simulink model "GATE_A"  (R2016a)
settings: Solver=FixedStepDiscrete  StartTime=0.0  StopTime=120  RelTol=1e-3
values from neighbouring files (symbols this model uses):
  CLOSE_CHAR = CHAR_STAR    [GateParameter.m]
  CLOSE_SIDE_VALUE = single(4*ONE_SEC)    [GateParameter.m]
  CLOSED = uint8(12)    [GateParameter.m]
  CLOSING = uint8(13)    [GateParameter.m]
  INIT = uint8(15)    [GateParameter.m]
  NO_PASS_ASSIG = uint8(6)    [GateParameter.m]
  OPEN = uint8(14)    [GateParameter.m]
  OPEN_CHAR = CHAR_HASH    [GateParameter.m]
  OPEN_SIDE_VALUE = uint16(4*ONE_SEC)    [GateParameter.m]
  OPENING = uint8(11)    [GateParameter.m]
  OPENING_ACTIVE = uint8(1)    [GateParameter.m]
  PASS_ASSIGNED = uint8(7)    [GateParameter.m]
  PASS_INCOMPLETE = uint8(8)    [GateParameter.m]
  PASS_TIMEOUT = uint16(10*ONE_SEC)    [GateParameter.m]
  PASSWORD_VERIFIED = uint8(5)    [GateParameter.m]
  TIMEOUT = uint8(9)    [GateParameter.m]
  WRONG_PASSWORD = uint8(2)    [GateParameter.m]
undefined symbols (not defined in the file or in its folder): OPEN_TIMEOUT
(part 1 of 2)
settings Model: ExtModeTrigDuration=2  Creator=omaro  LastModifiedBy=oelkawok
settings DataIOCC: SaveFormat=StructureWithTime  SaveOutput=off  SaveTime=off
settings OptimizationCC: DefaultParameterBehavior=Inlined  StateBitsets=on  DataBitsets=on  LifeSpan=1  MaxStackSize=64
settings DebuggingCC: ConsistencyChecking=error  SignalInfNanChecking=error  SignalRangeChecking=error  ReadBeforeWriteMsg=EnableAllAsError  WriteAfterWriteMsg=EnableAllAsError  WriteAfterReadMsg=EnableAllAsError  AlgebraicLoopMsg=error  ArtificialAlgebraicLoopMsg=error  BlockPriorityViolationMsg=error  MinStepSizeMsg=error  CheckMatrixSingularityMsg=error  ParameterUnderflowMsg=error  ParameterPrecisionLossMsg=error  UnderSpecifiedDataTypeMsg=warning  UnnecessaryDatatypeConvMsg=warning  VectorMatrixConversionMsg=error  SignalLabelMismatchMsg=error  UnconnectedInputMsg=error  UnconnectedOutputMsg=error  UnconnectedLineMsg=error  SFcnCompatibilityMsg=error  UniqueDataStoreMsg=error  BusObjectLabelMismatch=error  RootOutportRequireBusObject=error  ModelReferenceIOMsg=error  ModelReferenceVersionMismatchMessage=warning  ModelReferenceIOMismatchMessage=error  ModelReferenceDataLoggingMessage=error  StrictBusMsg=ErrorOnBusTreatedAsVector  SFUnusedDataAndEventsDiag=error  SFUnexpectedBacktrackingDiag=error  SFInvalidInputDataAccessInChartInitDiag=error  SFNoUnconditionalDefaultTransitionDiag=error  SFTransitionOutsideNaturalParentDiag=error  SFUndirectedBroadcastEventsDiag=error  SFTransitionActionBeforeConditionDiag=error  SFOutputUsedAsStateInMooreChartDiag=warning
settings HardwareCC: ProdBitPerInt=16  ProdBitPerPointer=16  ProdLargestAtomicFloat=None  ProdWordSize=8  ProdHWDeviceType=Atmel->AVR
settings SFSimCC: SimCustomHeaderCode=|
  | //#include "C:\Users\omaro\Desktop\Gate_Model\Arduino\Arduino.h"
  | //#include "Keypad\Keypad.h"
settings RTWCC: SystemTargetFile=ert.tlc  TemplateMakefile=ert_default_tmf  GenerateReport=on  RTWUseSimCustomCode=on  Toolchain=Arduino AVR v1.6.1  BuildConfiguration=Faster Runs  LaunchReport=on
settings RTWCC: CustomHeaderCode=|
  | //#include "C:\Users\omaro\Desktop\Gate_Model\Arduino\Arduino.h"
  | //#include "Keypad\Keypad.h"
settings CodeAppCC: ForceParamTrailComments=on  OperatorAnnotations=on  MATLABSourceComments=on
settings ERTTargetCC: ERTCustomFileBanners=off  SupportContinuousTime=on  SupportNonInlinedSFcns=on  SupportVariableSizeSignals=on  ModelStepFunctionPrototypeControlCompliant=off  RootIOFormat=Structure reference  ERTCustomFileTemplate=example_file_process.tlc

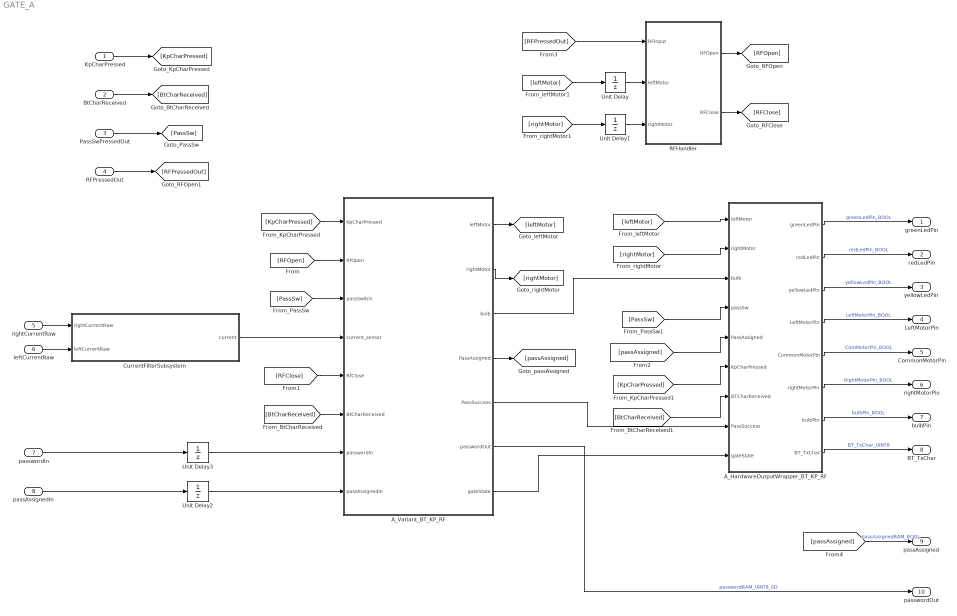
== system GATE_A ==
  KpCharPressed : Inport  OutDataTypeStr=uint8  PortDimensions=1  SampleTime=0
  BtCharReceived : Inport  Port=2  OutDataTypeStr=uint8  PortDimensions=1  SampleTime=0
  PassSwPressedOut : Inport  Port=3  OutDataTypeStr=boolean  PortDimensions=1  SampleTime=0
  RFPressedOut : Inport  Port=4  OutDataTypeStr=uint8  PortDimensions=1  SampleTime=0
  rightCurrentRaw : Inport  Port=5  OutDataTypeStr=uint16  PortDimensions=1  SampleTime=0
  leftCurrentRaw : Inport  Port=6  OutDataTypeStr=uint16  PortDimensions=1  SampleTime=0
  passwordIn : Inport  Port=7  OutDataTypeStr=uint8  PortDimensions=6  SampleTime=0
  passAssignedIn : Inport  Port=8  OutDataTypeStr=boolean  PortDimensions=1  SampleTime=0
  A_HardwareOutputWrapper_BT_KP_RF : Subsystem  VariantControl=Variant1
  A_Variant_BT_KP_RF : Subsystem  VariantControl=Variant
  CurrentFilterSubsystem : Subsystem
  RFHandler : Subsystem
  Unit Delay{,1..3} (4 alike) : UnitDelay  SampleTime=-1
  greenLedPin : Outport  OutDataTypeStr=boolean  PortDimensions=1  SampleTime=[0.001,0]
  redLedPin : Outport  Port=2  OutDataTypeStr=boolean  PortDimensions=1  SampleTime=[0.001,0]
  yellowLedPin : Outport  Port=3  OutDataTypeStr=boolean  PortDimensions=1  SampleTime=[0.001,0]
  LeftMotorPin : Outport  Port=4  OutDataTypeStr=boolean  PortDimensions=1  SampleTime=[0.001,0]
  CommonMotorPin : Outport  Port=5  OutDataTypeStr=boolean  PortDimensions=1  SampleTime=[0.001,0]
  rightMotorPin : Outport  Port=6  OutDataTypeStr=boolean  PortDimensions=1  SampleTime=[0.001,0]
  bulbPin : Outport  Port=7  OutDataTypeStr=boolean  PortDimensions=1  SampleTime=[0.001,0]
  BT_TxChar : Outport  Port=8  OutDataTypeStr=uint8  PortDimensions=1  SampleTime=[0.001,0]
  passAssigned : Outport  Port=9  OutDataTypeStr=boolean  PortDimensions=1  SampleTime=[0.001,0]
  passwordOut : Outport  Port=10  OutDataTypeStr=uint8  PortDimensions=6  SampleTime=[0.001,0]
  wires:
  RFHandler/1(RFOpen) -> [RFOpen]
  RFHandler/2(RFClose) -> [RFClose]
  [RFPressedOut] -> RFHandler/1(RFInput)
  RFPressedOut/1 -> [RFPressedOut]
  PassSwPressedOut/1 -> [PassSw]
  [leftMotor] -> Unit Delay/1
  Unit Delay/1 -> RFHandler/2(leftMotor)
  [rightMotor] -> Unit Delay1/1
  Unit Delay1/1 -> RFHandler/3(rightMotor)
  BtCharReceived/1 -> [BtCharReceived]
  KpCharPressed/1 -> [KpCharPressed]
  [RFOpen] -> A_Variant_BT_KP_RF/2(RfOpen)
  [PassSw] -> A_Variant_BT_KP_RF/3(passSwitch)
  [RFClose] -> A_Variant_BT_KP_RF/5(RfClose)
  [BtCharReceived] -> A_Variant_BT_KP_RF/6(BtCharReceived)
  A_Variant_BT_KP_RF/1(leftMotor) -> [leftMotor]
  A_Variant_BT_KP_RF/2(rightMotor) -> [rightMotor]
  [KpCharPressed] -> A_Variant_BT_KP_RF/1(KpCharPressed)
  [leftMotor] -> A_HardwareOutputWrapper_BT_KP_RF/1(leftMotor)
  [rightMotor] -> A_HardwareOutputWrapper_BT_KP_RF/2(rightMotor)
  A_Variant_BT_KP_RF/3(bulb) -> A_HardwareOutputWrapper_BT_KP_RF/3(bulb)
  [PassSw] -> A_HardwareOutputWrapper_BT_KP_RF/4(passSw)
  [KpCharPressed] -> A_HardwareOutputWrapper_BT_KP_RF/6(KpCharPressed)
  [BtCharReceived] -> A_HardwareOutputWrapper_BT_KP_RF/7(BTCharReceived)
  A_HardwareOutputWrapper_BT_KP_RF/1(greenLedPin) -> greenLedPin/1  "greenLedPin_BOOL"
  A_HardwareOutputWrapper_BT_KP_RF/2(redLedPin) -> redLedPin/1  "redLedPin_BOOL"
  A_HardwareOutputWrapper_BT_KP_RF/3(yellowLedPin) -> yellowLedPin/1  "yellowLedPin_BOOL"
  A_HardwareOutputWrapper_BT_KP_RF/4(LeftMotorPin) -> LeftMotorPin/1  "LeftMotorPin_BOOL"
  A_HardwareOutputWrapper_BT_KP_RF/5(CommonMotorPin) -> CommonMotorPin/1  "ComMotorPin_BOOL"
  A_HardwareOutputWrapper_BT_KP_RF/6(rightMotorPin) -> rightMotorPin/1  "RightMotorPin_BOOL"
  A_HardwareOutputWrapper_BT_KP_RF/7(bulbPin) -> bulbPin/1  "bulbPin_BOOL"
  A_HardwareOutputWrapper_BT_KP_RF/8(BT_TxChar) -> BT_TxChar/1  "BT_TxChar_UINT8"
  A_Variant_BT_KP_RF/4(PassAssigned) -> [passAssigned]
  [passAssigned] -> A_HardwareOutputWrapper_BT_KP_RF/5(PassAssigned)
  Unit Delay2/1 -> A_Variant_BT_KP_RF/8(passAssignedIn)
  Unit Delay3/1 -> A_Variant_BT_KP_RF/7(passwordIn)
  A_Variant_BT_KP_RF/5(PassSuccess) -> A_HardwareOutputWrapper_BT_KP_RF/8(PassSuccess)
  CurrentFilterSubsystem/1(current) -> A_Variant_BT_KP_RF/4(current_sensor)
  rightCurrentRaw/1 -> CurrentFilterSubsystem/1(rightCurrentRaw)
  leftCurrentRaw/1 -> CurrentFilterSubsystem/2(leftCurrentRaw)
  passAssignedIn/1 -> Unit Delay2/1
  passwordIn/1 -> Unit Delay3/1
  A_Variant_BT_KP_RF/6(passwordOut) -> passwordOut/1  "passwordRAM_UINT8_6D"
  [passAssigned] -> passAssigned/1  "passAssignedRAM_BOOL"
  A_Variant_BT_KP_RF/7(gateState) -> A_HardwareOutputWrapper_BT_KP_RF/9(gateState)

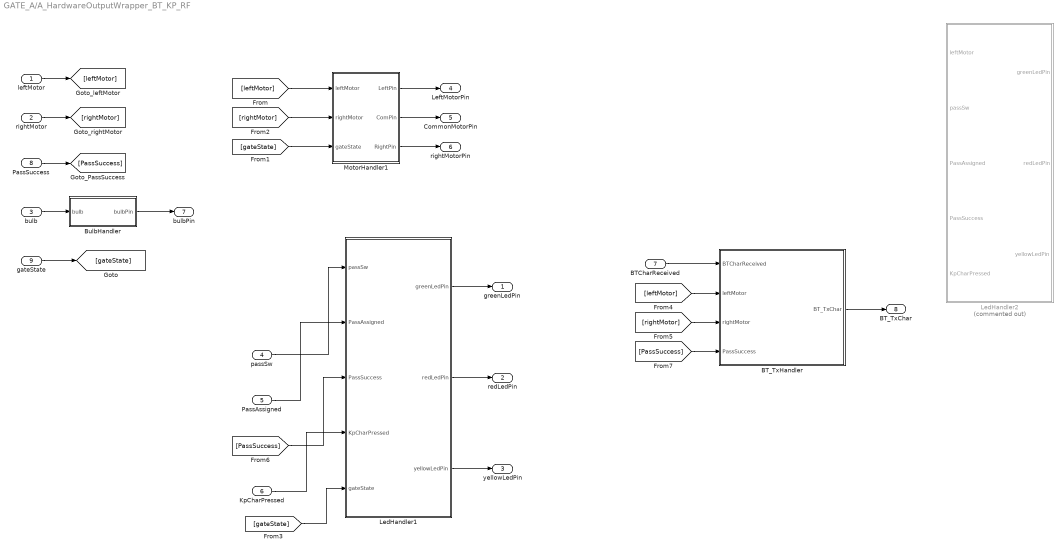
== system GATE_A/A_HardwareOutputWrapper_BT_KP_RF ==
  leftMotor : Inport
  rightMotor : Inport  Port=2
  bulb : Inport  Port=3
  passSw : Inport  Port=4
  PassAssigned : Inport  Port=5
  KpCharPressed : Inport  Port=6
  BTCharReceived : Inport  Port=7
  PassSuccess : Inport  Port=8
  gateState : Inport  Port=9
  BT_TxHandler : Subsystem
  BulbHandler : Subsystem
  LedHandler1 : Subsystem
  LedHandler2 : Subsystem  Commented=on
  MotorHandler1 : Subsystem
  greenLedPin : Outport
  redLedPin : Outport  Port=2
  yellowLedPin : Outport  Port=3
  LeftMotorPin : Outport  Port=4
  CommonMotorPin : Outport  Port=5
  rightMotorPin : Outport  Port=6
  bulbPin : Outport  Port=7
  BT_TxChar : Outport  Port=8
  wires:
  gateState/1 -> [gateState]
  [gateState] -> LedHandler1/5(gateState)
  [gateState] -> MotorHandler1/3(gateState)
  [leftMotor] -> MotorHandler1/1(leftMotor)
  BT_TxHandler/1(BT_TxChar) -> BT_TxChar/1
  [PassSuccess] -> BT_TxHandler/4(PassSuccess)
  PassSuccess/1 -> [PassSuccess]
  [rightMotor] -> BT_TxHandler/3(rightMotor)
  BTCharReceived/1 -> BT_TxHandler/1(BTCharReceived)
  [leftMotor] -> BT_TxHandler/2(leftMotor)
  KpCharPressed/1 -> LedHandler1/4(KpCharPressed)
  [PassSuccess] -> LedHandler1/3(PassSuccess)
  PassAssigned/1 -> LedHandler1/2(PassAssigned)
  passSw/1 -> LedHandler1/1(passSw)
  rightMotor/1 -> [rightMotor]
  leftMotor/1 -> [leftMotor]
  BulbHandler/1(bulbPin) -> bulbPin/1
  MotorHandler1/3(RightPin) -> rightMotorPin/1
  MotorHandler1/2(ComPin) -> CommonMotorPin/1
  MotorHandler1/1(LeftPin) -> LeftMotorPin/1
  LedHandler1/3(yellowLedPin) -> yellowLedPin/1
  LedHandler1/2(redLedPin) -> redLedPin/1
  LedHandler1/1(greenLedPin) -> greenLedPin/1
  bulb/1 -> BulbHandler/1(bulb)
  [rightMotor] -> MotorHandler1/2(rightMotor)

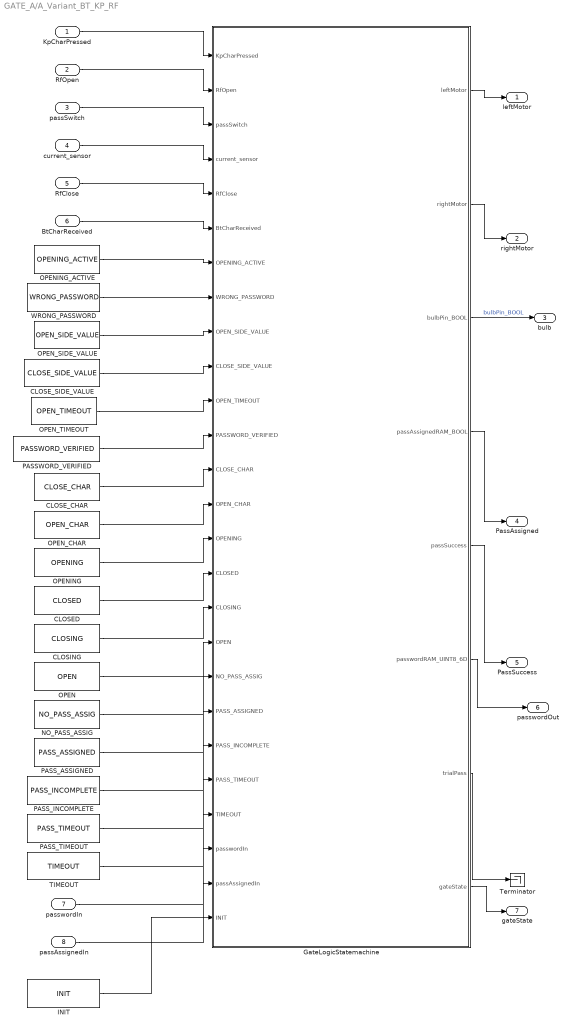
== system GATE_A/A_Variant_BT_KP_RF ==
  KpCharPressed : Inport
  RfOpen : Inport  Port=2
  passSwitch : Inport  Port=3
  current_sensor : Inport  Port=4
  RfClose : Inport  Port=5
  BtCharReceived : Inport  Port=6
  passwordIn : Inport  Port=7
  passAssignedIn : Inport  Port=8
  CLOSED : Constant  Value=CLOSED  SampleTime=-1
  CLOSE_CHAR : Constant  Value=CLOSE_CHAR  SampleTime=-1
  CLOSE_SIDE_VALUE : Constant  Value=CLOSE_SIDE_VALUE  SampleTime=-1
  CLOSING : Constant  Value=CLOSING  SampleTime=-1
  GateLogicStatemachine : Stateflow chart  TreatAsAtomicUnit=on
  INIT : Constant  Value=INIT  SampleTime=-1
  NO_PASS_ASSIG : Constant  Value=NO_PASS_ASSIG  SampleTime=-1
  OPEN : Constant  Value=OPEN  SampleTime=-1
  OPENING : Constant  Value=OPENING  SampleTime=-1
  OPENING_ACTIVE : Constant  Value=OPENING_ACTIVE  SampleTime=-1
  OPEN_CHAR : Constant  Value=OPEN_CHAR  SampleTime=-1
  OPEN_SIDE_VALUE : Constant  Value=OPEN_SIDE_VALUE  SampleTime=-1
  OPEN_TIMEOUT : Constant  Value=OPEN_TIMEOUT  SampleTime=-1
  PASSWORD_VERIFIED : Constant  Value=PASSWORD_VERIFIED  SampleTime=-1
  PASS_ASSIGNED : Constant  Value=PASS_ASSIGNED  SampleTime=-1
  PASS_INCOMPLETE : Constant  Value=PASS_INCOMPLETE  SampleTime=-1
  PASS_TIMEOUT : Constant  Value=PASS_TIMEOUT  SampleTime=-1
  TIMEOUT : Constant  Value=TIMEOUT  SampleTime=-1
  Terminator : Terminator
  WRONG_PASSWORD : Constant  Value=WRONG_PASSWORD  SampleTime=-1
  leftMotor : Outport
  rightMotor : Outport  Port=2
  bulb : Outport  Port=3
  PassAssigned : Outport  Port=4
  PassSuccess : Outport  Port=5
  passwordOut : Outport  Port=6
  gateState : Outport  Port=7
  wires:
  GateLogicStatemachine/8(gateState) -> gateState/1
  INIT/1 -> GateLogicStatemachine/26(INIT)
  GateLogicStatemachine/7(trialPass) -> Terminator/1
  passAssignedIn/1 -> GateLogicStatemachine/25(passAssignedIn)
  passwordIn/1 -> GateLogicStatemachine/24(passwordIn)
  GateLogicStatemachine/6(passwordRAM_UINT8_6D) -> passwordOut/1
  CLOSING/1 -> GateLogicStatemachine/17(CLOSING)
  OPENING/1 -> GateLogicStatemachine/15(OPENING)
  CLOSED/1 -> GateLogicStatemachine/16(CLOSED)
  OPEN_CHAR/1 -> GateLogicStatemachine/14(OPEN_CHAR)
  CLOSE_CHAR/1 -> GateLogicStatemachine/13(CLOSE_CHAR)
  OPEN/1 -> GateLogicStatemachine/18(OPEN)
  PASSWORD_VERIFIED/1 -> GateLogicStatemachine/12(PASSWORD_VERIFIED)
  RfOpen/1 -> GateLogicStatemachine/2(RfOpen)
  GateLogicStatemachine/3(bulbPin_BOOL) -> bulb/1  "bulbPin_BOOL"
  current_sensor/1 -> GateLogicStatemachine/4(current_sensor)
  WRONG_PASSWORD/1 -> GateLogicStatemachine/8(WRONG_PASSWORD)
  GateLogicStatemachine/1(leftMotor) -> leftMotor/1
  GateLogicStatemachine/2(rightMotor) -> rightMotor/1
  OPENING_ACTIVE/1 -> GateLogicStatemachine/7(OPENING_ACTIVE)
  OPEN_SIDE_VALUE/1 -> GateLogicStatemachine/9(OPEN_SIDE_VALUE)
  OPEN_TIMEOUT/1 -> GateLogicStatemachine/11(OPEN_TIMEOUT)
  CLOSE_SIDE_VALUE/1 -> GateLogicStatemachine/10(CLOSE_SIDE_VALUE)
  NO_PASS_ASSIG/1 -> GateLogicStatemachine/19(NO_PASS_ASSIG)
  BtCharReceived/1 -> GateLogicStatemachine/6(BtCharReceived)
  KpCharPressed/1 -> GateLogicStatemachine/1(KpCharPressed)
  PASS_TIMEOUT/1 -> GateLogicStatemachine/22(PASS_TIMEOUT)
  GateLogicStatemachine/5(passSuccess) -> PassSuccess/1
  passSwitch/1 -> GateLogicStatemachine/3(passSwitch)
  GateLogicStatemachine/4(passAssignedRAM_BOOL) -> PassAssigned/1
  PASS_ASSIGNED/1 -> GateLogicStatemachine/20(PASS_ASSIGNED)
  PASS_INCOMPLETE/1 -> GateLogicStatemachine/21(PASS_INCOMPLETE)
  TIMEOUT/1 -> GateLogicStatemachine/23(TIMEOUT)
  RfClose/1 -> GateLogicStatemachine/5(RfClose)

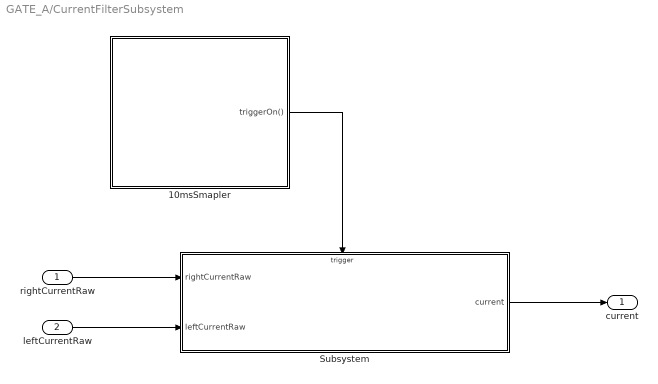
== system GATE_A/CurrentFilterSubsystem ==
  rightCurrentRaw : Inport
  leftCurrentRaw : Inport  Port=2
  10msSmapler : Stateflow chart  TreatAsAtomicUnit=on
  Subsystem : Subsystem
  current : Outport
  wires:
  leftCurrentRaw/1 -> Subsystem/2(leftCurrentRaw)
  rightCurrentRaw/1 -> Subsystem/1(rightCurrentRaw)
  Subsystem/1(current) -> current/1
  10msSmapler/1(triggerOn()) -> Subsystem/Trigger

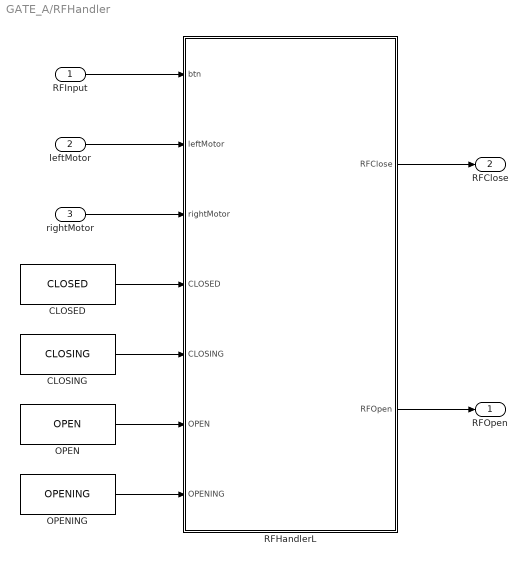
== system GATE_A/RFHandler ==
  RFInput : Inport
  leftMotor : Inport  Port=2
  rightMotor : Inport  Port=3
  CLOSED : Constant  Value=CLOSED  SampleTime=-1
  CLOSING : Constant  Value=CLOSING  SampleTime=-1
  OPEN : Constant  Value=OPEN  SampleTime=-1
  OPENING : Constant  Value=OPENING  SampleTime=-1
  RFHandlerL : Stateflow chart  TreatAsAtomicUnit=on
  RFOpen : Outport
  RFClose : Outport  Port=2
  wires:
  rightMotor/1 -> RFHandlerL/3(rightMotor)
  leftMotor/1 -> RFHandlerL/2(leftMotor)
  OPENING/1 -> RFHandlerL/7(OPENING)
  CLOSED/1 -> RFHandlerL/4(CLOSED)
  CLOSING/1 -> RFHandlerL/5(CLOSING)
  OPEN/1 -> RFHandlerL/6(OPEN)
  RFHandlerL/2(RFOpen) -> RFOpen/1
  RFHandlerL/1(RFClose) -> RFClose/1
  RFInput/1 -> RFHandlerL/1(btn)

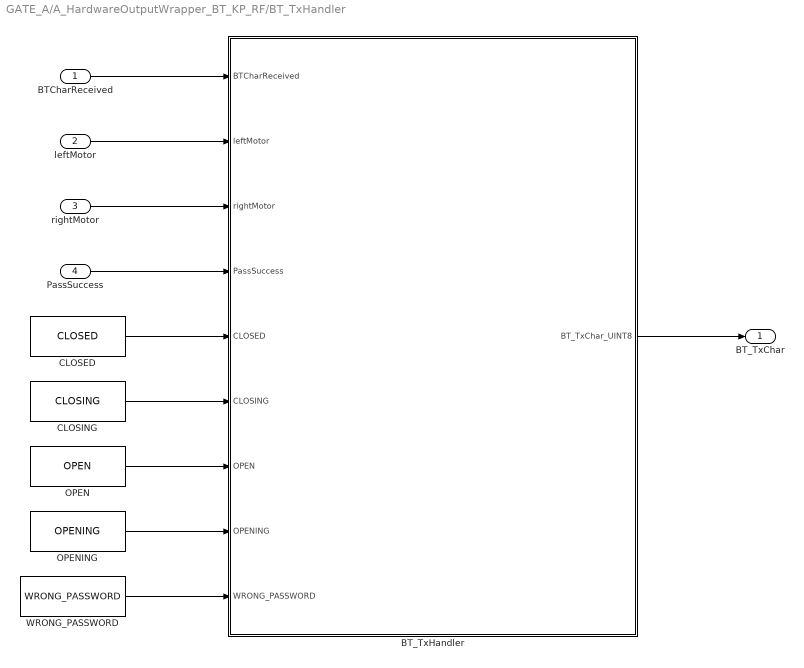
== system GATE_A/A_HardwareOutputWrapper_BT_KP_RF/BT_TxHandler ==
  BTCharReceived : Inport
  leftMotor : Inport  Port=2
  rightMotor : Inport  Port=3
  PassSuccess : Inport  Port=4
  BT_TxHandler : Stateflow chart  TreatAsAtomicUnit=on
  CLOSED : Constant  Value=CLOSED  SampleTime=-1
  CLOSING : Constant  Value=CLOSING  SampleTime=-1
  OPEN : Constant  Value=OPEN  SampleTime=-1
  OPENING : Constant  Value=OPENING  SampleTime=-1
  WRONG_PASSWORD : Constant  Value=WRONG_PASSWORD  SampleTime=-1
  BT_TxChar : Outport
  wires:
  WRONG_PASSWORD/1 -> BT_TxHandler/9(WRONG_PASSWORD)
  OPENING/1 -> BT_TxHandler/8(OPENING)
  OPEN/1 -> BT_TxHandler/7(OPEN)
  CLOSING/1 -> BT_TxHandler/6(CLOSING)
  CLOSED/1 -> BT_TxHandler/5(CLOSED)
  PassSuccess/1 -> BT_TxHandler/4(PassSuccess)
  BT_TxHandler/1(BT_TxChar_UINT8) -> BT_TxChar/1
  rightMotor/1 -> BT_TxHandler/3(rightMotor)
  leftMotor/1 -> BT_TxHandler/2(leftMotor)
  BTCharReceived/1 -> BT_TxHandler/1(BTCharReceived)

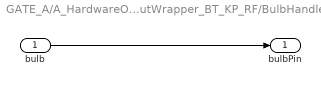
== system GATE_A/A_HardwareOutputWrapper_BT_KP_RF/BulbHandler ==
  bulb : Inport
  bulbPin : Outport
  wires:
  bulb/1 -> bulbPin/1

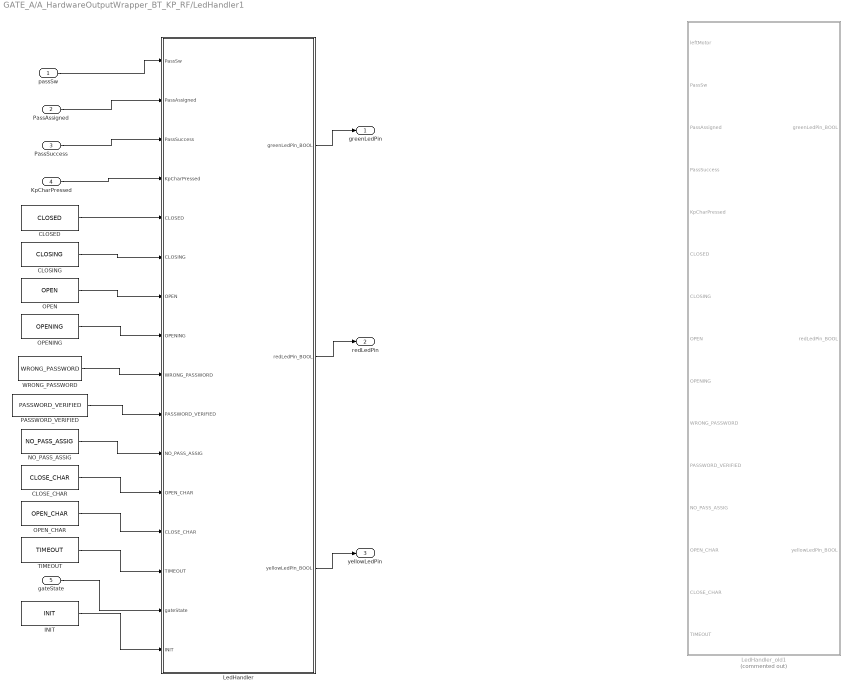
== system GATE_A/A_HardwareOutputWrapper_BT_KP_RF/LedHandler1 ==
  passSw : Inport
  PassAssigned : Inport  Port=2
  PassSuccess : Inport  Port=3
  KpCharPressed : Inport  Port=4
  gateState : Inport  Port=5
  CLOSED : Constant  Value=CLOSED  SampleTime=-1
  CLOSE_CHAR : Constant  Value=CLOSE_CHAR  SampleTime=-1
  CLOSING : Constant  Value=CLOSING  SampleTime=-1
  INIT : Constant  Value=INIT  SampleTime=-1
  LedHandler : Stateflow chart  TreatAsAtomicUnit=on
  LedHandler_old1 : Stateflow chart  Commented=on  TreatAsAtomicUnit=on
  NO_PASS_ASSIG : Constant  Value=NO_PASS_ASSIG  SampleTime=-1
  OPEN : Constant  Value=OPEN  SampleTime=-1
  OPENING : Constant  Value=OPENING  SampleTime=-1
  OPEN_CHAR : Constant  Value=OPEN_CHAR  SampleTime=-1
  PASSWORD_VERIFIED : Constant  Value=PASSWORD_VERIFIED  SampleTime=-1
  TIMEOUT : Constant  Value=TIMEOUT  SampleTime=-1
  WRONG_PASSWORD : Constant  Value=WRONG_PASSWORD  SampleTime=-1
  greenLedPin : Outport
  redLedPin : Outport  Port=2
  yellowLedPin : Outport  Port=3
  wires:
  LedHandler/1(greenLedPin_BOOL) -> greenLedPin/1
  LedHandler/2(redLedPin_BOOL) -> redLedPin/1
  LedHandler/3(yellowLedPin_BOOL) -> yellowLedPin/1
  passSw/1 -> LedHandler/1(PassSw)
  PassAssigned/1 -> LedHandler/2(PassAssigned)
  PassSuccess/1 -> LedHandler/3(PassSuccess)
  OPENING/1 -> LedHandler/8(OPENING)
  OPEN/1 -> LedHandler/7(OPEN)
  CLOSING/1 -> LedHandler/6(CLOSING)
  CLOSED/1 -> LedHandler/5(CLOSED)
  WRONG_PASSWORD/1 -> LedHandler/9(WRONG_PASSWORD)
  PASSWORD_VERIFIED/1 -> LedHandler/10(PASSWORD_VERIFIED)
  NO_PASS_ASSIG/1 -> LedHandler/11(NO_PASS_ASSIG)
  KpCharPressed/1 -> LedHandler/4(KpCharPressed)
  CLOSE_CHAR/1 -> LedHandler/12(OPEN_CHAR)
  OPEN_CHAR/1 -> LedHandler/13(CLOSE_CHAR)
  TIMEOUT/1 -> LedHandler/14(TIMEOUT)
  gateState/1 -> LedHandler/15(gateState)
  INIT/1 -> LedHandler/16(INIT)

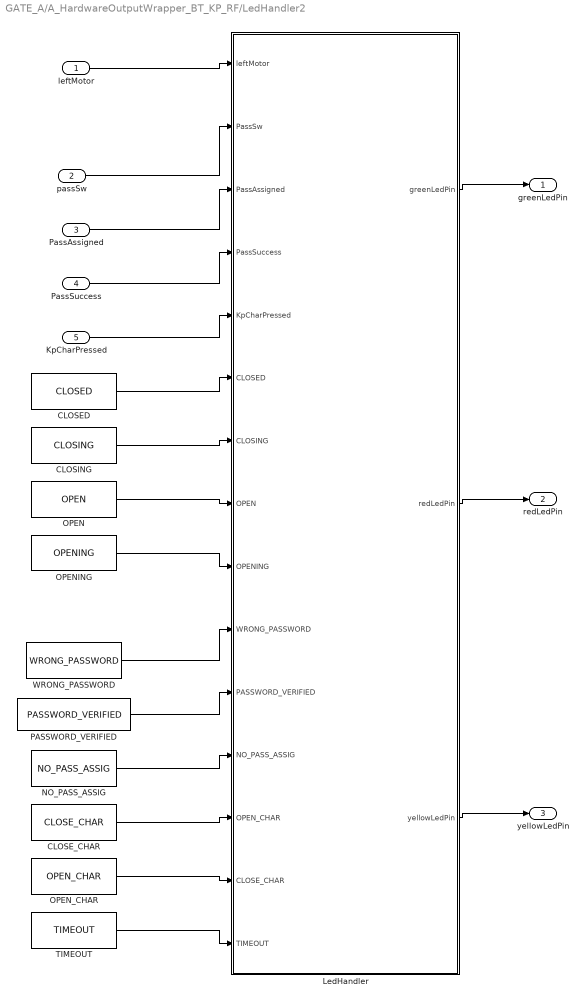
== system GATE_A/A_HardwareOutputWrapper_BT_KP_RF/LedHandler2 ==
  leftMotor : Inport
  passSw : Inport  Port=2
  PassAssigned : Inport  Port=3
  PassSuccess : Inport  Port=4
  KpCharPressed : Inport  Port=5
  CLOSED : Constant  Value=CLOSED  SampleTime=-1
  CLOSE_CHAR : Constant  Value=CLOSE_CHAR  SampleTime=-1
  CLOSING : Constant  Value=CLOSING  SampleTime=-1
  LedHandler : Stateflow chart  TreatAsAtomicUnit=on
  NO_PASS_ASSIG : Constant  Value=NO_PASS_ASSIG  SampleTime=-1
  OPEN : Constant  Value=OPEN  SampleTime=-1
  OPENING : Constant  Value=OPENING  SampleTime=-1
  OPEN_CHAR : Constant  Value=OPEN_CHAR  SampleTime=-1
  PASSWORD_VERIFIED : Constant  Value=PASSWORD_VERIFIED  SampleTime=-1
  TIMEOUT : Constant  Value=TIMEOUT  SampleTime=-1
  WRONG_PASSWORD : Constant  Value=WRONG_PASSWORD  SampleTime=-1
  greenLedPin : Outport
  redLedPin : Outport  Port=2
  yellowLedPin : Outport  Port=3
  wires:
  leftMotor/1 -> LedHandler/1(leftMotor)
  LedHandler/1(greenLedPin) -> greenLedPin/1
  LedHandler/2(redLedPin) -> redLedPin/1
  LedHandler/3(yellowLedPin) -> yellowLedPin/1
  passSw/1 -> LedHandler/2(PassSw)
  PassAssigned/1 -> LedHandler/3(PassAssigned)
  PassSuccess/1 -> LedHandler/4(PassSuccess)
  OPENING/1 -> LedHandler/9(OPENING)
  OPEN/1 -> LedHandler/8(OPEN)
  CLOSING/1 -> LedHandler/7(CLOSING)
  CLOSED/1 -> LedHandler/6(CLOSED)
  WRONG_PASSWORD/1 -> LedHandler/10(WRONG_PASSWORD)
  PASSWORD_VERIFIED/1 -> LedHandler/11(PASSWORD_VERIFIED)
  NO_PASS_ASSIG/1 -> LedHandler/12(NO_PASS_ASSIG)
  KpCharPressed/1 -> LedHandler/5(KpCharPressed)
  CLOSE_CHAR/1 -> LedHandler/13(OPEN_CHAR)
  OPEN_CHAR/1 -> LedHandler/14(CLOSE_CHAR)
  TIMEOUT/1 -> LedHandler/15(TIMEOUT)

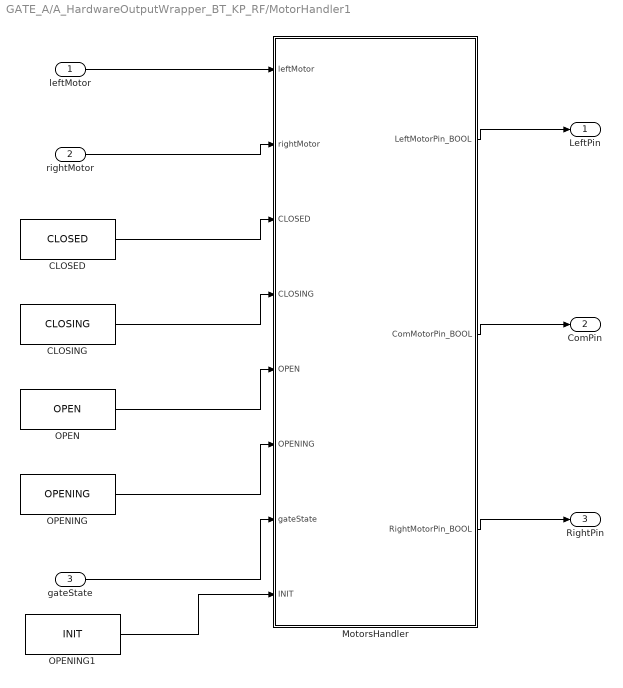
== system GATE_A/A_HardwareOutputWrapper_BT_KP_RF/MotorHandler1 ==
  leftMotor : Inport
  rightMotor : Inport  Port=2
  gateState : Inport  Port=3
  CLOSED : Constant  Value=CLOSED  SampleTime=-1
  CLOSING : Constant  Value=CLOSING  SampleTime=-1
  MotorsHandler : Stateflow chart  TreatAsAtomicUnit=on
  OPEN : Constant  Value=OPEN  SampleTime=-1
  OPENING : Constant  Value=OPENING  SampleTime=-1
  OPENING1 : Constant  Value=INIT  SampleTime=-1
  LeftPin : Outport
  ComPin : Outport  Port=2
  RightPin : Outport  Port=3
  wires:
  rightMotor/1 -> MotorsHandler/2(rightMotor)
  CLOSED/1 -> MotorsHandler/3(CLOSED)
  CLOSING/1 -> MotorsHandler/4(CLOSING)
  OPEN/1 -> MotorsHandler/5(OPEN)
  OPENING/1 -> MotorsHandler/6(OPENING)
  MotorsHandler/1(LeftMotorPin_BOOL) -> LeftPin/1
  MotorsHandler/2(ComMotorPin_BOOL) -> ComPin/1
  MotorsHandler/3(RightMotorPin_BOOL) -> RightPin/1
  gateState/1 -> MotorsHandler/7(gateState)
  leftMotor/1 -> MotorsHandler/1(leftMotor)
  OPENING1/1 -> MotorsHandler/8(INIT)

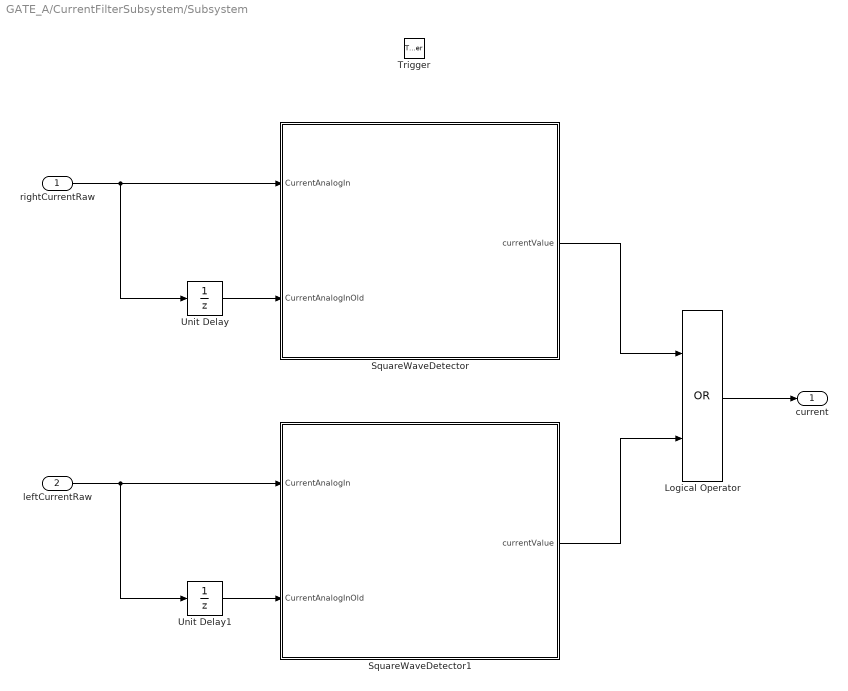
== system GATE_A/CurrentFilterSubsystem/Subsystem ==
  rightCurrentRaw : Inport
  leftCurrentRaw : Inport  Port=2
  Trigger : TriggerPort  TriggerType=function-call  VariantControl=Variant  PortDimensions=1
  Logical Operator : Logic  Operator=OR  AllPortsSameDT=off  OutDataTypeStr=boolean
  SquareWaveDetector : Stateflow chart  TreatAsAtomicUnit=on
  SquareWaveDetector1 : Stateflow chart  TreatAsAtomicUnit=on
  Unit Delay : UnitDelay  SampleTime=-1
  Unit Delay1 : UnitDelay  SampleTime=-1
  current : Outport
  wires:
  Logical Operator/1 -> current/1
  SquareWaveDetector1/1(currentValue) -> Logical Operator/2
  SquareWaveDetector/1(currentValue) -> Logical Operator/1
  Unit Delay1/1 -> SquareWaveDetector1/2(CurrentAnalogInOld)
  leftCurrentRaw/1 -> SquareWaveDetector1/1(CurrentAnalogIn), Unit Delay1/1
  Unit Delay/1 -> SquareWaveDetector/2(CurrentAnalogInOld)
  rightCurrentRaw/1 -> Unit Delay/1, SquareWaveDetector/1(CurrentAnalogIn)

== stateflow chart GATE_A/A_HardwareOutputWrapper_BT_KP_RF/LedHandler2/LedHandler ==
  state AssigningPass
    en:
    counter = 0;
    state Start
      en:
      yellowLedPin = true;
      greenLedPin = false;
      redLedPin = false;
    state correctPassAssigned
      du:
      counter++;
    state incorrectPassAssigned
      du:
      counter++;
    (default) -> AssigningPass.Start
    AssigningPass.Start -> correctPassAssigned [order 1] : [PassAssigned == true]/greenLedPin = true;
    AssigningPass.Start -> incorrectPassAssigned [order 2] : [(PassSw == false) && (PassAssigned == false)]
        | /redLedPin = true;...
        | yellowLedPin = false;
    correctPassAssigned -> correctPassAssigned : [(hasChanged(PassSw)) ...
        | && (PassSw == false)]
        | /yellowLedPin = false;
  state EnteringPass
    en:
    counter = 0;
    state correctPass
      en:
      yellowLedPin = false;
      greenLedPin = true;
      redLedPin = false;
      du:
      counter++;
    state Start
    state IncorrectPass
      en:
      yellowLedPin = false;
      greenLedPin = false;
      redLedPin = true;
      du:
      counter++;
    EnteringPass.Start -> correctPass [order 1] : [PassSuccess == PASSWORD_VERIFIED]
    (default) -> EnteringPass.Start
    EnteringPass.Start -> IncorrectPass [order 2] : [(PassSuccess == TIMEOUT)...
        |  || (PassSuccess == WRONG_PASSWORD)]
  state Idle
    en:
    yellowLedPin = false;
    greenLedPin = false;
    redLedPin = false;
  state GateOn
    en:
    yellowLedPin = false;
    greenLedPin = true;
    redLedPin = false;
  (default) -> Idle
  EnteringPass -> Idle [order 2] : [PassSuccess == NO_PASS_ASSIG]
  Idle -> AssigningPass [order 1] : [PassSw == true]
  correctPass -> Idle : [counter >= 4800]
  AssigningPass -> Idle [order 1] : [(counter >= 4900)]
  Idle -> EnteringPass [order 2] : [(hasChanged(KpCharPressed)) ...
      | && (KpCharPressed != 0)...
      | && (KpCharPressed != OPEN_CHAR)...
      | && (KpCharPressed != CLOSE_CHAR)...
      | && (PassAssigned == true)]
      | /yellowLedPin = true;
  IncorrectPass -> Idle : [counter >= 4800]
  Idle -> GateOn [order 3] : [(leftMotor == OPENING)...
      |  || (leftMotor == OPEN)...
      |  || (leftMotor == CLOSING)]
  GateOn -> Idle : [leftMotor == CLOSED]
  EnteringPass -> GateOn [order 1] : [(leftMotor == OPENING)...
      | || (leftMotor == OPEN)...
      | || (leftMotor == CLOSING)]
  AssigningPass -> GateOn [order 2] : [(leftMotor == OPENING)...
      |  || (leftMotor == OPEN)...
      |  || (leftMotor == CLOSING)]
  data: leftMotor input; greenLedPin output boolean =false; redLedPin output boolean =false; yellowLedPin output boolean =false; PassSw input; counter local uint16; PassAssigned input; PassSuccess input; KpCharPressed input; CLOSED input; CLOSING input; OPEN input; OPENING input; WRONG_PASSWORD input; PASSWORD_VERIFIED input; NO_PASS_ASSIG input; OPEN_CHAR input; CLOSE_CHAR input; TIMEOUT input

== stateflow chart GATE_A/CurrentFilterSubsystem/10msSmapler ==
  (default) -> (junction 2)
  (junction 2) -> (junction 3) : {counter_1ms++;}
  (junction 3) -> (junction 6) : [counter_1ms == 10]
      | {
      | triggerOn;
      | counter_1ms = 0;
      | }
  data: counter_1ms local double
  events: triggerOn output FUNCTION_CALL_EVENT

== stateflow chart GATE_A/CurrentFilterSubsystem/Subsystem/SquareWaveDetector ==
  state Running
    entry:
    counterHigh = 0;
    counterLow= 0;
    currentValue = 1;
    state High
      entry:
      counterLow = 0;
    state Low
      entry:
      counterHigh = 0;
    (default) -> High
    High -> High [order 2] : [CurrentAnalogIn > 1000]
        | /counterHigh++;
    High -> Low [order 1] : [CurrentAnalogIn < 1000]
    Low -> High [order 1] : [CurrentAnalogIn > 1000]
    Low -> Low [order 2] : [CurrentAnalogIn < 1000]
        | /counterLow++
  state Stop
    entry:
    currentValue = 0;
    stableCounter = 0;
    state PosEdge
    state NegEdge
    (default) -> PosEdge
    PosEdge -> NegEdge : [(CurrentAnalogInOld > 1000)...
        |  && (CurrentAnalogIn < 1000)]...
        | /stableCounter += 1;
    NegEdge -> PosEdge : [(CurrentAnalogInOld < 1000)...
        |  && (CurrentAnalogIn > 1000)]...
        | /stableCounter += 1;
  (default) -> Stop
  Stop -> Running : [(CurrentAnalogInOld != CurrentAnalogIn) && stableCounter > 2]
  Running -> Stop : [(counterHigh >= 50)...
      |  || (counterLow >= 50)]
  data: CurrentAnalogIn input; currentValue output uint8; counterHigh local uint16; counterLow local uint16; stableCounter local uint8; CurrentAnalogInOld input

== stateflow chart GATE_A/CurrentFilterSubsystem/Subsystem/SquareWaveDetector1 ==
  state Running
    entry:
    counterHigh = 0;
    counterLow= 0;
    currentValue = 1;
    state High
      entry:
      counterLow = 0;
    state Low
      entry:
      counterHigh = 0;
    (default) -> High
    High -> High [order 2] : [CurrentAnalogIn > 1000]
        | /counterHigh++;
    High -> Low [order 1] : [CurrentAnalogIn < 1000]
    Low -> High [order 1] : [CurrentAnalogIn > 1000]
    Low -> Low [order 2] : [CurrentAnalogIn < 1000]
        | /counterLow++
  state Stop
    entry:
    currentValue = 0;
    stableCounter = 0;
    state PosEdge
    state NegEdge
    (default) -> PosEdge
    PosEdge -> NegEdge : [(CurrentAnalogInOld > 1000)...
        |  && (CurrentAnalogIn < 1000)]...
        | /stableCounter += 1;
    NegEdge -> PosEdge : [(CurrentAnalogInOld < 1000)...
        |  && (CurrentAnalogIn > 1000)]...
        | /stableCounter += 1;
  (default) -> Stop
  Stop -> Running : [(CurrentAnalogInOld != CurrentAnalogIn) && stableCounter > 2]
  Running -> Stop : [(counterHigh >= 50)...
      |  || (counterLow >= 50)]
  data: CurrentAnalogIn input; currentValue output uint8; counterHigh local uint16; counterLow local uint16; stableCounter local uint8; CurrentAnalogInOld input

== stateflow chart GATE_A/RFHandler/RFHandlerL ==
  state Close
    entry:
    RFOpen = false;
    RFClose = true;
  state RFOff
    entry:
    RFOpen = false;
    RFClose = false;
  state Open
    entry:
    RFOpen = true;
    RFClose = false;
    counter = 0;
    du:
    counter++;
  Close -> RFOff [order 1] : [rightMotor == CLOSED]
  Close -> (junction 11) [order 2] : [hasChanged(btn)]
  (junction 11) -> Close [order 2] : [(btn == 1) ...
      | && ((leftMotor == OPENING)...
      | || (leftMotor == OPEN))]
  (default) -> RFOff
  RFOff -> (junction 11) : [hasChanged(btn)]
  Open -> (junction 11) [order 2] : [hasChanged(btn)]
  (junction 11) -> Open [order 1] : [(btn == 1) ...
      | && ((leftMotor == CLOSING)...
      | || (leftMotor == CLOSED))]
  Open -> RFOff [order 1] : [(counter == 5) ...
      | && ((leftMotor == CLOSING)...
      | || (leftMotor == CLOSED))]
  data: btn input; RFClose output boolean; RFOpen output boolean; leftMotor input; rightMotor input; CLOSED input; CLOSING input; OPEN input; OPENING input; counter local uint8

== stateflow chart GATE_A/A_Variant_BT_KP_RF/GateLogicStatemachine ==
  state opening
    entry:
    bulbPin_BOOL = true;
    gateState = OPENING;
    state openLeftSide
      entry:
      leftMotor = OPENING;
      openSideDelay = 0;
      during:
      openSideDelay++;
    state openRightSide
      entry:
      rightMotor = OPENING;
    (default) -> openLeftSide
    openLeftSide -> openRightSide : [openSideDelay == OPEN_SIDE_VALUE]
  state init
    entry:
    passSuccess = NO_PASS_ASSIG;
    gotoReady = false;
    bulbPin_BOOL = 0;
    leftMotor = CLOSED;
    rightMotor = CLOSED;
    gateState = INIT;
    state idle
      entry:
      passAssignedRAM_BOOL = false;
    state AssignPass
      entry:
      counter = 0;
      state addToPass
        entry:
        passwordRAM_UINT8_6D[counter] = KpCharPressed;
      state MonitoringNumber
      state PassAssigned
        entry:
        gotoReady = true;
      (junction 259) -> addToPass : [KpCharPressed != 0]
      MonitoringNumber -> (junction 259) [order 1] : [hasChanged(KpCharPressed)]
      (default) -> MonitoringNumber
      addToPass -> MonitoringNumber [order 1] : [counter < 5]/counter++;
      MonitoringNumber -> PassAssigned [order 2] : [RfOpen == true]
      addToPass -> PassAssigned [order 2] : [counter == 5]
          | / passAssignedRAM_BOOL = true;...
          | passSuccess = PASS_ASSIGNED;
    state PassAssignedPreviously
      entry:
      passwordRAM_UINT8_6D[0] = passwordIn[0];
      passwordRAM_UINT8_6D[1] = passwordIn[1];
      passwordRAM_UINT8_6D[2] = passwordIn[2];
      passwordRAM_UINT8_6D[3] = passwordIn[3];
      passwordRAM_UINT8_6D[4] = passwordIn[4];
      passwordRAM_UINT8_6D[5] = passwordIn[5];
      passAssignedRAM_BOOL = passAssignedIn;
      gotoReady = true;
    (default) -> idle
    idle -> AssignPass [order 1] : [passSwitch==true]
    idle -> PassAssignedPreviously [order 2] : [passAssignedIn]
    AssignPass -> idle : [passSwitch==false]
  state closed
    entry:
    bulbPin_BOOL = false;
    leftMotor = CLOSED;
    rightMotor = CLOSED;
    openingActive = 0;
    gateState = CLOSED;
    state BTPassHandler
      state monitorBtnPressed
      state btnPressed
        entry:
        trialPass[counter] = BtCharReceived;
      state initTrailPass
        entry:
        initCounter = 1;
        state initiatePass
          entry:
          trialPass[initCounter] = 0;
        (junction 295) -> closed.BTPassHandler.initTrailPass.initiatePass
        (default) -> (junction 295)
        closed.BTPassHandler.initTrailPass.initiatePass -> (junction 295) : [initCounter < 5]...
            | /initCounter++;
      state verifyPass
        (default) -> (junction 301)
        (junction 301) -> (junction 302) [order 1] : [trialPass[0] != passwordRAM_UINT8_6D[0]]
        (junction 301) -> (junction 303) [order 2]
        (junction 302) -> (junction 319) : {passSuccess = WRONG_PASSWORD;}
        (junction 303) -> (junction 304) [order 1] : [trialPass[1] != passwordRAM_UINT8_6D[1]]
        (junction 303) -> (junction 305) [order 2]
        (junction 304) -> (junction 318) : {passSuccess = WRONG_PASSWORD;}
        (junction 305) -> (junction 306) [order 1] : [trialPass[2] != passwordRAM_UINT8_6D[2]]
        (junction 305) -> (junction 307) [order 2]
        (junction 306) -> (junction 317) : {passSuccess = WRONG_PASSWORD;}
        (junction 307) -> (junction 308) [order 1] : [trialPass[3] != passwordRAM_UINT8_6D[3]]
        (junction 307) -> (junction 309) [order 2]
        (junction 308) -> (junction 316) : {passSuccess = WRONG_PASSWORD;}
        (junction 309) -> (junction 310) [order 1] : [trialPass[4] != passwordRAM_UINT8_6D[4]]
        (junction 309) -> (junction 311) [order 2]
        (junction 310) -> (junction 315) : {passSuccess = WRONG_PASSWORD;}
        (junction 311) -> (junction 312) [order 1] : [trialPass[5] != passwordRAM_UINT8_6D[5]]
        (junction 311) -> (junction 313) [order 2] : {passSuccess = PASSWORD_VERIFIED;}
        (junction 312) -> (junction 314) : {passSuccess = WRONG_PASSWORD;}
        (junction 314) -> (junction 313)
        (junction 315) -> (junction 314)
        (junction 316) -> (junction 315)
        (junction 317) -> (junction 316)
        (junction 318) -> (junction 317)
        (junction 319) -> (junction 318)
        (junction 313) -> (junction 320)
      (default) -> closed.BTPassHandler.initTrailPass
      closed.BTPassHandler.monitorBtnPressed -> (junction 277) : [hasChanged...
          | (BtCharReceived)]
      (junction 277) -> closed.BTPassHandler.btnPressed : [BtCharReceived != 0]/{counter++;}
      closed.BTPassHandler.initTrailPass -> closed.BTPassHandler.monitorBtnPressed : [initCounter == 5]...
          | /{counter = 0;}
      closed.BTPassHandler.btnPressed -> closed.BTPassHandler.monitorBtnPressed [order 1] : [counter < 5]
      (junction 279) -> closed.BTPassHandler.initTrailPass
      closed.BTPassHandler.btnPressed -> closed.BTPassHandler.verifyPass [order 2] : [counter >= 5]
      closed.BTPassHandler.verifyPass -> (junction 279) : [(passSuccess == PASSWORD_VERIFIED)]
          | / {openingActive = OPENING_ACTIVE;}
    state openingGate
    state MonitorInput
      entry:
      passTimer = 0;
    state KpPassHandler
      du:
      passTimer++;
      state monitorBtnPressed
      state btnPressed
        entry:
        trialPass[counter] = KpCharPressed;
      state initTrailPass
        entry:
        initCounter = 1;
        state initiatePass
          entry:
          trialPass[initCounter] = 0;
        (junction 269) -> closed.KpPassHandler.initTrailPass.initiatePass
        (default) -> (junction 269)
        closed.KpPassHandler.initTrailPass.initiatePass -> (junction 269) : [initCounter < 5]...
            | /initCounter++;
      state verifyPass
        (default) -> (junction 115)
        (junction 115) -> (junction 116) [order 1] : [trialPass[0] != passwordRAM_UINT8_6D[0]]
        (junction 115) -> (junction 119) [order 2]
        (junction 116) -> (junction 118) : {passSuccess = WRONG_PASSWORD;}
        (junction 119) -> (junction 122) [order 1] : [trialPass[1] != passwordRAM_UINT8_6D[1]]
        (junction 119) -> (junction 120) [order 2]
        (junction 122) -> (junction 121) : {passSuccess = WRONG_PASSWORD;}
        (junction 120) -> (junction 144) [order 1] : [trialPass[2] != passwordRAM_UINT8_6D[2]]
        (junction 120) -> (junction 143) [order 2]
        (junction 144) -> (junction 168) : {passSuccess = WRONG_PASSWORD;}
        (junction 143) -> (junction 149) [order 1] : [trialPass[3] != passwordRAM_UINT8_6D[3]]
        (junction 143) -> (junction 153) [order 2]
        (junction 149) -> (junction 169) : {passSuccess = WRONG_PASSWORD;}
        (junction 153) -> (junction 156) [order 1] : [trialPass[4] != passwordRAM_UINT8_6D[4]]
        (junction 153) -> (junction 157) [order 2]
        (junction 156) -> (junction 170) : {passSuccess = WRONG_PASSWORD;}
        (junction 157) -> (junction 158) [order 1] : [trialPass[5] != passwordRAM_UINT8_6D[5]]
        (junction 157) -> (junction 164) [order 2] : {passSuccess = PASSWORD_VERIFIED;}
        (junction 158) -> (junction 171) : {passSuccess = WRONG_PASSWORD;}
        (junction 171) -> (junction 164)
        (junction 170) -> (junction 171)
        (junction 169) -> (junction 170)
        (junction 168) -> (junction 169)
        (junction 121) -> (junction 168)
        (junction 118) -> (junction 121)
        (junction 164) -> (junction 165)
      (default) -> closed.KpPassHandler.initTrailPass
      closed.KpPassHandler.monitorBtnPressed -> (junction 263) : [hasChanged...
          | (KpCharPressed)]
      (junction 263) -> closed.KpPassHandler.btnPressed : [KpCharPressed != 0]/{counter++;}
      closed.KpPassHandler.initTrailPass -> closed.KpPassHandler.monitorBtnPressed : [initCounter == 5]...
          | /{counter = 0;}
      closed.KpPassHandler.btnPressed -> closed.KpPassHandler.monitorBtnPressed [order 1] : [counter < 5]
      (junction 262) -> closed.KpPassHandler.initTrailPass : [(KpCharPressed == OPEN_CHAR)...
          |  && (KpCharPressed != 0)]...
          |  / {openingActive = OPENING_ACTIVE;}
      closed.KpPassHandler.btnPressed -> closed.KpPassHandler.verifyPass [order 2] : [counter >= 5]
      closed.KpPassHandler.verifyPass -> (junction 262) : [hasChanged(KpCharPressed) && (passSuccess == PASSWORD_VERIFIED)]
    (junction 350) -> BTPassHandler : [(BtCharReceived != 0) ...
        | && passAssignedRAM_BOOL]
        | /passSuccess = PASS_INCOMPLETE;...
        | trialPass[0] = BtCharReceived;
    MonitorInput -> (junction 350) [order 3] : [hasChanged...
        | (BtCharReceived)]
    BTPassHandler -> openingGate [order 2] : [openingActive == OPENING_ACTIVE]
    BTPassHandler -> MonitorInput [order 1] : [passSuccess == WRONG_PASSWORD]
    MonitorInput -> openingGate [order 1] : [RfOpen]/{openingActive = OPENING_ACTIVE;}
    (default) -> MonitorInput
    KpPassHandler -> MonitorInput [order 3] : [(passTimer == PASS_TIMEOUT)]
        | /passSuccess = TIMEOUT;
    KpPassHandler -> openingGate [order 1] : [openingActive == OPENING_ACTIVE]
    MonitorInput -> (junction 260) [order 2] : [hasChanged...
        | (KpCharPressed)]
    KpPassHandler -> MonitorInput [order 2] : [(passSuccess == WRONG_PASSWORD)]
    (junction 260) -> KpPassHandler : [(KpCharPressed != 0) ...
        | &&(KpCharPressed != OPEN_CHAR)...
        | &&(KpCharPressed != CLOSE_CHAR)...
        | && passAssignedRAM_BOOL]
        | /passSuccess = PASS_INCOMPLETE;...
        | trialPass[0] = KpCharPressed;
  state closing
    entry:
    gateState = CLOSING;
    state closingRightSide
      entry:
      rightMotor = CLOSING;
      closeSideDelay = 0;
      during:
      closeSideDelay++;
    state closingLeftSide
      entry:
      leftMotor = CLOSING;
    (default) -> closingRightSide
    closingRightSide -> closingLeftSide : [closeSideDelay == CLOSE_SIDE_VALUE]
  state open
    entry:
    gateState = OPEN;
    state gateOpen
      entry:
      closing_active = false;
      leftMotor = OPEN;
      rightMotor = OPEN;
      openTimer = 0;
      du:
      openTimer++;
    state closing
      entry:
      closing_active = true;
    (default) -> gateOpen
    gateOpen -> (junction 264) [order 1] : [hasChanged(KpCharPressed)]
    (junction 264) -> open.closing : [(KpCharPressed == CLOSE_CHAR)]
    gateOpen -> (junction 355) [order 3] : [hasChanged(BtCharReceived)]
    (junction 355) -> open.closing : [BtCharReceived == CLOSE_CHAR]
    gateOpen -> open.closing [order 2] : [RfClose]
    gateOpen -> open.closing [order 4] : [openTimer == OPEN_TIMEOUT]
  closed -> (junction 258) [order 1] : [hasChanged(passSwitch)]
  (junction 258) -> init : [passSwitch]
  (default) -> init
  init -> closed [order 1] : [gotoReady == true]
  closed -> opening [order 2] : [openingActive == OPENING_ACTIVE]
  init -> closed [order 2] : [RfOpen == true]
  closing -> closed : [(current_sensor == 0)...
      | &&(leftMotor == CLOSING)...
      | &&(rightMotor == CLOSING)]
  opening -> open : [(current_sensor == 0)...
      | && (leftMotor == OPENING)...
      | && (rightMotor == OPENING)]
  open -> closing : [closing_active == true]
  data: KpCharPressed input; RfOpen input; openingActive local uint8; passSwitch input; counter local uint8; closing_active local uint8; current_sensor input; initCounter local uint8; openSideDelay local uint16; leftMotor output uint8 =0; rightMotor output uint8 =0; bulbPin_BOOL output boolean; RfClose input; closeSideDelay local uint16; BtCharReceived input; OPENING_ACTIVE input =2; WRONG_PASSWORD input =1; OPEN_SIDE_VALUE input =20; CLOSE_SIDE_VALUE input =20; OPEN_TIMEOUT input =999999; PASSWORD_VERIFIED input =3; CLOSE_CHAR input =12; OPEN_CHAR input; OPENING input =2; CLOSED input =1; CLOSING input =4; OPEN input =3; passAssignedRAM_BOOL output boolean; gotoReady local boolean; passSuccess output uint8 =0; NO_PASS_ASSIG input; PASS_ASSIGNED input; PASS_INCOMPLETE input; PASS_TIMEOUT input; passTimer local uint16; TIMEOUT input; openTimer local uint16; passwordRAM_UINT8_6D output uint8 size=6; passwordIn input size=6; passAssignedIn input; trialPass output uint8 size=6; INIT input; gateState output uint8

== stateflow chart GATE_A/A_HardwareOutputWrapper_BT_KP_RF/LedHandler1/LedHandler_old1 ==
  state AssigningPass
    en:
    counter = 0;
    state Start
      en:
      yellowLedPin_BOOL = true;
      greenLedPin_BOOL = false;
      redLedPin_BOOL = false;
    state correctPassAssigned
      du:
      counter++;
    state incorrectPassAssigned
      du:
      counter++;
    (default) -> AssigningPass.Start
    AssigningPass.Start -> correctPassAssigned [order 1] : [PassAssigned == true]/greenLedPin_BOOL = true;
    AssigningPass.Start -> incorrectPassAssigned [order 2] : [(PassSw == false) && (PassAssigned == false)]
        | /redLedPin_BOOL = true;...
        | yellowLedPin_BOOL = false;
    correctPassAssigned -> correctPassAssigned : [(hasChanged(PassSw)) ...
        | && (PassSw == false)]
        | /yellowLedPin_BOOL = false;
  state EnteringPass
    en:
    counter = 0;
    state correctPass
      en:
      yellowLedPin_BOOL = false;
      greenLedPin_BOOL = true;
      redLedPin_BOOL = false;
      du:
      counter++;
    state Start
    state IncorrectPass
      en:
      yellowLedPin_BOOL = false;
      greenLedPin_BOOL = false;
      redLedPin_BOOL = true;
      du:
      counter++;
    EnteringPass.Start -> correctPass [order 1] : [PassSuccess == PASSWORD_VERIFIED]
    (default) -> EnteringPass.Start
    EnteringPass.Start -> IncorrectPass [order 2] : [(PassSuccess == TIMEOUT)...
        |  || (PassSuccess == WRONG_PASSWORD)]
  state Idle
    en:
    yellowLedPin_BOOL = false;
    greenLedPin_BOOL = false;
    redLedPin_BOOL = false;
  state GateOn
    en:
    yellowLedPin_BOOL = false;
    greenLedPin_BOOL = true;
    redLedPin_BOOL = false;
  (default) -> Idle
  EnteringPass -> Idle [order 2] : [PassSuccess == NO_PASS_ASSIG]
  Idle -> AssigningPass [order 1] : [PassSw == true]
  correctPass -> Idle : [counter >= 4800]
  AssigningPass -> Idle [order 1] : [(counter >= 4900)]
  Idle -> EnteringPass [order 2] : [(hasChanged(KpCharPressed)) ...
      | && (KpCharPressed != 0)...
      | && (KpCharPressed != OPEN_CHAR)...
      | && (KpCharPressed != CLOSE_CHAR)...
      | && (PassAssigned == true)]
      | /yellowLedPin_BOOL = true;
  IncorrectPass -> Idle : [counter >= 4800]
  Idle -> GateOn [order 3] : [(leftMotor == OPENING)...
      |  || (leftMotor == OPEN)...
      |  || (leftMotor == CLOSING)]
  GateOn -> Idle : [leftMotor == CLOSED]
  EnteringPass -> GateOn [order 1] : [(leftMotor == OPENING)...
      | || (leftMotor == OPEN)...
      | || (leftMotor == CLOSING)]
  AssigningPass -> GateOn [order 2] : [(leftMotor == OPENING)...
      |  || (leftMotor == OPEN)...
      |  || (leftMotor == CLOSING)]
  data: leftMotor input; greenLedPin_BOOL output boolean =false; redLedPin_BOOL output boolean =false; yellowLedPin_BOOL output boolean =false; PassSw input; counter local uint16; PassAssigned input; PassSuccess input; KpCharPressed input; CLOSED input; CLOSING input; OPEN input; OPENING input; WRONG_PASSWORD input; PASSWORD_VERIFIED input; NO_PASS_ASSIG input; OPEN_CHAR input; CLOSE_CHAR input; TIMEOUT input

== stateflow chart GATE_A/A_HardwareOutputWrapper_BT_KP_RF/LedHandler1/LedHandler ==
  state AssigningPass
    state Start
      en:
      counter = 0;
      yellowLedPin_BOOL = true;
      greenLedPin_BOOL = false;
      redLedPin_BOOL = false;
    state correctPassAssigned
      du:
      counter++;
    state incorrectPassAssigned
      du:
      counter++;
    (default) -> AssigningPass.Start
    AssigningPass.Start -> incorrectPassAssigned [order 2] : [(PassSw == false) && (PassAssigned == false)]
        | /redLedPin_BOOL = true;...
        | yellowLedPin_BOOL = false;
    AssigningPass.Start -> correctPassAssigned [order 1] : [PassAssigned == true]/greenLedPin_BOOL = true;
    correctPassAssigned -> correctPassAssigned : [(hasChanged(PassSw)) ...
        | && (PassSw == false)]
        | /yellowLedPin_BOOL = false;
  state EnteringPass
    en:
    counter = 0;
    state correctPass
      en:
      yellowLedPin_BOOL = false;
      greenLedPin_BOOL = true;
      redLedPin_BOOL = false;
      du:
      counter++;
    state Start
    state IncorrectPass
      en:
      yellowLedPin_BOOL = false;
      greenLedPin_BOOL = false;
      redLedPin_BOOL = true;
      du:
      counter++;
    EnteringPass.Start -> correctPass [order 1] : [PassSuccess == PASSWORD_VERIFIED]
    (default) -> EnteringPass.Start
    EnteringPass.Start -> IncorrectPass [order 2] : [(PassSuccess == TIMEOUT)...
        |  || (PassSuccess == WRONG_PASSWORD)]
  state Idle
    en:
    counter = 0;
    yellowLedPin_BOOL = false;
    greenLedPin_BOOL = false;
    redLedPin_BOOL = false;
  state GateOn
    en:
    yellowLedPin_BOOL = false;
    greenLedPin_BOOL = true;
    redLedPin_BOOL = false;
  (default) -> Idle
  EnteringPass -> Idle [order 2] : [PassSuccess == NO_PASS_ASSIG]
  Idle -> AssigningPass [order 1] : [PassSw == true]
  correctPass -> (junction 113)
  AssigningPass -> Idle [order 1] : [(counter >= 4900)]
  Idle -> (junction 113) [order 3]
  (junction 113) -> Idle [order 1] : [counter >= 4800]
  Idle -> GateOn [order 2] : [(gateState == OPENING)...
      |  || (gateState == OPEN)...
      |  || (gateState == CLOSING)]
  GateOn -> Idle : [gateState == CLOSED]
  (junction 113) -> EnteringPass [order 2] : [(hasChanged(KpCharPressed)) ...
      | && (KpCharPressed != 0)...
      | && (KpCharPressed != OPEN_CHAR)...
      | && (KpCharPressed != CLOSE_CHAR)...
      | && (PassAssigned == true)...
      | && (gateState != INIT)]
      | /yellowLedPin_BOOL = true;
      | greenLedPin_BOOL = false;
      | redLedPin_BOOL = false;
  IncorrectPass -> (junction 113)
  EnteringPass -> GateOn [order 1] : [(gateState == OPENING)...
      | || (gateState == OPEN)...
      | || (gateState == CLOSING)]
  AssigningPass -> GateOn [order 2] : [(gateState == OPENING)...
      |  || (gateState == OPEN)...
      |  || (gateState == CLOSING)]
  AssigningPass -> AssigningPass [order 3] : [hasChanged(PassSw) ...
      | && PassSw == true]
  data: greenLedPin_BOOL output boolean =false; redLedPin_BOOL output boolean =false; yellowLedPin_BOOL output boolean =false; PassSw input; counter local uint16; PassAssigned input; PassSuccess input; KpCharPressed input; CLOSED input; CLOSING input; OPEN input; OPENING input; WRONG_PASSWORD input; PASSWORD_VERIFIED input; NO_PASS_ASSIG input; OPEN_CHAR input; CLOSE_CHAR input; TIMEOUT input; gateState input; INIT input

== stateflow chart GATE_A/A_HardwareOutputWrapper_BT_KP_RF/MotorHandler1/MotorsHandler ==
  state MonitorChange
  state UpdatePins
    (default) -> (junction 91) : /* updating motor Pins Switch case */
    (junction 91) -> (junction 92) [order 1] : [(leftMotor == OPENING) && ((rightMotor == CLOSED) || (rightMotor == OPEN))]
    (junction 92) -> (junction 100) : {LeftMotorPin_BOOL = true;...
        | ComMotorPin_BOOL = true;...
        | RightMotorPin_BOOL = false;}
    (junction 91) -> (junction 93) [order 2]
    (junction 93) -> (junction 94) [order 1] : [(leftMotor == CLOSING) && ((rightMotor == CLOSED) || (rightMotor == OPEN))]
    (junction 94) -> (junction 99) : {LeftMotorPin_BOOL = false;...
        | ComMotorPin_BOOL = false;...
        |  RightMotorPin_BOOL = true;}
    (junction 93) -> (junction 95) [order 2]
    (junction 95) -> (junction 96) [order 1] : [(rightMotor == CLOSING) && ((leftMotor == CLOSED) || (leftMotor == OPEN))]
    (junction 96) -> (junction 98) : {LeftMotorPin_BOOL = true;...
        | ComMotorPin_BOOL = false;...
        | RightMotorPin_BOOL = false;}
    (junction 95) -> (junction 102) [order 2]
    (junction 102) -> (junction 103) [order 1] : [(rightMotor == OPENING) && ((leftMotor == CLOSED) || (leftMotor == OPEN))]
    (junction 103) -> (junction 110) : {LeftMotorPin_BOOL = false;...
        | ComMotorPin_BOOL = true;...
        | RightMotorPin_BOOL = true;}
    (junction 102) -> (junction 104) [order 2]
    (junction 104) -> (junction 105) [order 1] : [(rightMotor == OPENING) && (leftMotor == OPENING)]
    (junction 105) -> (junction 111) : {LeftMotorPin_BOOL = true;...
        | ComMotorPin_BOOL = true;...
        | RightMotorPin_BOOL = true;}
    (junction 104) -> (junction 106) [order 2]
    (junction 106) -> (junction 107) [order 1] : [(rightMotor == CLOSING) && (leftMotor == CLOSING)]
    (junction 106) -> (junction 123) [order 2]
    (junction 107) -> (junction 112) : {LeftMotorPin_BOOL = false;...
        | ComMotorPin_BOOL = false;...
        | RightMotorPin_BOOL = false;}
    (junction 123) -> (junction 124) [order 1] : [((rightMotor == CLOSED) || (rightMotor == OPEN)) ...
        | && ((leftMotor == CLOSED) || (leftMotor == OPEN))]
    (junction 123) -> (junction 136) [order 2]
    (junction 124) -> (junction 125) : {LeftMotorPin_BOOL = false;...
        | ComMotorPin_BOOL = true;...
        | RightMotorPin_BOOL = false;}
    (junction 136) -> (junction 138) [order 1] : [(gateState == CLOSED) || (gateState == OPEN) || (gateState == INIT)]
    (junction 136) -> (junction 97) [order 2]
    (junction 138) -> (junction 139) : {LeftMotorPin_BOOL = false;...
        | ComMotorPin_BOOL = true;...
        | RightMotorPin_BOOL = false;}
    (junction 100) -> (junction 99)
    (junction 99) -> (junction 98)
    (junction 98) -> (junction 110)
    (junction 139) -> (junction 97)
    (junction 125) -> (junction 139)
    (junction 112) -> (junction 125)
    (junction 111) -> (junction 112)
    (junction 110) -> (junction 111)
    (junction 97) -> (junction 101)
  (default) -> MonitorChange
  UpdatePins -> MonitorChange
  MonitorChange -> UpdatePins : [(hasChanged(leftMotor)) ...
      | || (hasChanged(rightMotor))...
      | || (hasChanged(gateState) && (gateState == CLOSED))...
      |  || (hasChanged(gateState) && (gateState == OPEN))...
      | ||(hasChanged(gateState) && (gateState == INIT))]
  data: leftMotor input; LeftMotorPin_BOOL output boolean =false; ComMotorPin_BOOL output boolean =true; RightMotorPin_BOOL output boolean =false; rightMotor input; CLOSED input; CLOSING input; OPEN input; OPENING input; gateState input; INIT input
